simulink model "Phil_VMP_DP_Combo_Task"  (R2013a)
settings: Solver=ode4  SolverMode=SingleTasking  StartTime=0.0  StopTime=inf  FixedStep=BKIN_STEP_TIME  RelTol=1e-3
StartFcn:
  |  warndlg('Dexterit-E models cannot run under simulation. Please compile your model and run it from within Dexterit-E.');set_param(bdroot,'SimulationCommand','stop')
model workspace (MAT data in the model file):
  col_x = 1
  col_y = 2
  RADIUS_VIS = 3
  COLOR_INIT = 4
  START_TARGET_COL = 1
  DELAY_POST_TRIAL_COL = 6
  MAX_REACH_TIME_COL = 4
  DELAY_COL = 5
  BKIN_STEP_TIME = 0.0005
  E_TRIAL_SUCCESS = 8
  SECOND_TARGET_COL = 3
  E_SECOND_TARGET_ON = 4
  WAIT_IN_HOME_COL = 2
  RADIUS_FUNC = 5
  E_SECOND_TARGET_REACHED = 5
  E_TRIAL_FAILURE = 7
  E_NEW_TRIAL = 3
  E_HOME_TARGET_REACHED = 2
  E_SHOW_HOME_TARGET = 6
  LOAD = 1
  TRIAL_TYPE_COL = 7
  RH_LOAD_COL = 8
  Cursor_Diameter_COL = 1
  SPEED_THRESHOLD_START = 2
  GOLDILOCKS = 6
  TOO_FAST = 8
  TOO_SLOW = 7
  LENGTH = 9
  WIDTH = 10
  ROTATION = 11
  SPEED_FEEDBACK_COL = 11
  GOLDILOCKS_COL = 12
  TOO_SLOW_COL = 13
  BASELINE_EEG_COL = 14
  BASELINE_DUR_COL = 15
  E_EEG_BASELINE = 1
  FORCE_CHANNEL_COL = 16
  WALL_WIDTH = 2
  CHANNEL_WIDTH = 3
  VISCOSITY = 4
  E_DEFINE_TRIAL_TYPE = 9
  CHANNEL_LOAD_COL = 17
  HAND_SPEED_THRESHOLD_COL = 18
  E_MOVEMENT_START = 10
  E_BASELINE_END = 11
  ROTATION_ANGLE_COL = 19
  VIS_VS_KIN_COL = 9
  DISTANCE_TO_HOME_COL = 10
  ROTATION_TYPE_COL = 20
  CONST_VISC_FORCE_COL = 21
  VISC_X = 5
  CURL_X = 6
  CURL_Y = 7
  VISC_Y = 8
undefined symbols (not defined in the file): Hand_Feedback, KINARM_DistanceFromTarget, KINARM_general, KINARM_HandInTarget, slselsubs
libraries: xpclib x6, KINARM_EP_loads x4, General x3, Video x3, xpcnilib x1
(part 3 of 3)

== matlab function Phil_VMP_DP_Combo_Task/Visual_Rotation/Triggered Subsystem/Embedded MATLAB Function ==
  settings: fimath=|
      | fimath(...
      | 'RoundMode', 'floor',...
      | 'OverflowMode', 'wrap',...
      | 'ProductMode', 'KeepLSB', 'ProductWordLength', 32,...
      | 'SumMode', 'KeepLSB', 'SumWordLength', 32,...
      | 'CastBeforeSum', false)
  data: rotation output; Trial_Protocol input
function rotation   = Calculate_Desired_Rotation(Trial_Protocol)
% This block supports an embeddable subset of the MATLAB language.
% See the help menu for details. 

%This block was modified by IEB, Sept 24, 2008
%It updates the desired amount of rotation

% NOTE ALL ROTATIONS ARE CURRENTLY IN DEGREES IN THE FUNCTION

% create a persistent variable to remember the rotation amount from one time-step to the next
persistent rotation_memory

if isempty(rotation_memory),            rotation_memory = 0;										end

% where to look in the TP table for these parameters
rotate_type_COL = 20;
rotation_amount_COL = 19;

rotate_type = Trial_Protocol(rotate_type_COL);
rotation_amount = Trial_Protocol(rotation_amount_COL);

if rotate_type == 0
	%set the rotation = 0
	rotation = 0;
elseif rotate_type ==1
	%set the rotation = specified amount
	rotation = rotation_amount;
elseif rotate_type == 2
	%set the rotation to change by specified amount
	rotation = rotation_memory + rotation_amount;
else
	%do nothing
	rotation = rotation_memory;
end

% save the rotation amount for the next time-step
rotation_memory = rotation;

== matlab function Phil_VMP_DP_Combo_Task/Create_MirrorTarget_Table/Embedded MATLAB Mirror Target Table ==
  settings: fimath=|
      | fimath(...
      | 'RoundMode', 'floor',...
      | 'OverflowMode', 'wrap',...
      | 'ProductMode', 'KeepLSB', 'ProductWordLength', 32,...
      | 'SumMode', 'KeepLSB', 'SumWordLength', 32,...
      | 'CastBeforeSum', false)
  data: shoulderXpos input size=2; Mirror_Target_Table output; Target_Table input; Midline_Target_Table output
function [Mirror_Target_Table,Midline_Target_Table]= FMirror_TT(shoulderXpos, Target_Table)
% this function creates a Mirror_Target_Table that is the mirror image of 
% the Target Table, flipped in the X-direction around the subject's midline
% The subject's midline is assumed to be halfway between the two shoulders.

% It also creates a midline Target Table with all targets on the midline.

% all dimensions in m unless otherwise stated
% arguments:
% shoulderXpos: x positions of shoulders (m)
% Target_Table: the complete Target_Table (cm in v1.4)


target_col_x = 1;
center_x = mean(shoulderXpos)*100;				%calculate the subject's midline position (cm)
Mirror_Target_Table = Target_Table;
Midline_Target_Table = Target_Table;

Mirror_Target_Table(:,target_col_x) = 2*center_x-Target_Table(:,target_col_x);
Midline_Target_Table(:,target_col_x) = center_x;

== matlab function Phil_VMP_DP_Combo_Task/Show_Mirror_Target/Embedded MATLAB Function ==
  settings: fimath=|
      | fimath(...
      | 'RoundMode', 'floor',...
      | 'OverflowMode', 'wrap',...
      | 'ProductMode', 'KeepLSB', 'ProductWordLength', 32,...
      | 'SumMode', 'KeepLSB', 'SumWordLength', 32,...
      | 'CastBeforeSum', false)
  data: target input; VCODE output; state input; target_type input; opacity input; target_display input; x_index input; y_index input; num_states input; stateindices input
function VCODE  = fcn(target, state, target_type, opacity, target_display, x_index, y_index, num_states, stateindices)

% VCODEs are length 70. All units in a VCODE should be SI, e.g. (m) and (rad). Elements in a VCODE are defined as follows:
%
% For all target types:
%  1: target type
%       1 - circle
%       2 - ellipse
%       3 - rectangle
%       4 - line
%       5 - triangle
%       11 - circle with label
%       12 - ellipse with label
%       13 - rectangle with label
%       14 - line with label
%       15 - triangle with label
%  2: target on/off status and target display (which display target will appear on)
%		0 - off
%		1 - on, appearing on both subject and operator displays
%       2 - on, appearing on subject display only
%       3 - on, appearing on operator display only
%  3: x position (m)
%  4: y position (m)
%  5: fill colour (RRGGBB) or texture index
%  6: stroke colour (RRGGBB) or texture index
%  7: stroke width
%  8: reserved for target background ID
%  9: opacity
%
% For circles:
%  10: radius (m)
%
% For ellipses:
%  10: major radius (m)
%  11: minor radius (m)
%  12: orientation of major axis (rad)
%
% For rectangles:
%  10: length (m)
%  11: height (m)
%  12: orientation (rad) (relative to x, y already shown)
%
% For lines:
%  10: endpoint x-axis coordinate relative to start point (m)
%  11: endpoint y-axis coordinate relative to start point (m)
%
% For triangles:
%  10: length (m)
%  11: height (m)
%  12: offset of peak from midpoint of length (m)
%  13: orientation (rad)
%
% For all labelled target types:
%  14: reserved
%  15-64: label characters (indexes in ISO 8859-1 character set)
%  65: label colour (0xRRGGBB), opacity is set by the vcode's opacity (9).
%  66: label height (m)
%  67: reserved
%  68: reserved
%  69: reserved
%  70: reserved

VCODE = zeros(1, 70);

% Set the target type.
VCODE(1) = target_type;

% Set the target on/off state. If the state input is 0, the target is off. Users of the VCODE should respect this
% as an indication that the rest of the VCODE will be uninitialized.
if (state <= 0) || (state > num_states)
	VCODE(2) = 0;  % target is off
	return;
else
	VCODE(2) = target_display;  % target is on; target displays as specified by block mask
end

% Set the target position.
VCODE(3) = target(x_index) * 0.01;  % x position (convert from (cm) in target table to (m))
VCODE(4) = target(y_index) * 0.01;  % y position (convert from (cm) in target table to (m))

% Set the fill colour. Fill colour currently comes from the GUI in RRRGGGBBB format.
if stateindices(state, 1) == 0
	VCODE(5) = -2^31;
elseif target(stateindices(state, 1)) < 0
    VCODE(5) = target(stateindices(state, 1));
else
	VCODE(5) = colourshift(target(stateindices(state, 1)));
end

% Set the stroke colour. Stroke colour currently comes from the GUI in RRRGGGBBB format.
if stateindices(state, 2) == 0
	VCODE(6) = -2^31;
elseif target(stateindices(state, 2)) < 0
    VCODE(6) = target(stateindices(state, 2));
else
	VCODE(6) = colourshift(target(stateindices(state, 2)));
end

% Set the stroke width. if target table index for stroke width is zero, then the stroke width is undefined
if stateindices(state, 3) == 0
	VCODE(7) = 0;                   % if stroke width column is 0, then stroke width is 0
elseif stateindices(state, 3) < 0
	VCODE(7) = 0.001;               % if stroke width column is -ve, then a 1mm default is chosen
else
	VCODE(7) = target(stateindices(state, 3)) * 0.01;  % if stroke width column is +ve, convert width from (cm) in target table to (m)
end

% Set the opacity value, clamping it to [0, 100].
if opacity <= 0
    VCODE(9) = 0.0;
elseif opacity >= 100
    VCODE(9) = 100.0;
else
    VCODE(9) = opacity;
end

% Set attributes specific to each target type.
if target_type == 1

    % Handle circle target:
	VCODE(10)=target(stateindices(state, 4)) * 0.01;  % radius (convert from (cm) in target table to (m))

elseif target_type == 2

    % Handle ellipse target:
	VCODE(10) = target(stateindices(state, 4)) * 0.01;  % major radius (convert from (cm) in target table to (m))
	VCODE(11) = target(stateindices(state, 5)) * 0.01;  % minor radius (convert from (cm) in target table to (m))

    if stateindices(state, 6) == 0
		VCODE(12) = 0;  % if orientation column is 0, set orientation to 0 rad
	else
		VCODE(12) = mod(target(stateindices(state, 6)), 360) * pi / 180.0;  % orientation (convert from (degrees) in target table to (rad))
    end

elseif target_type == 3

    % Handle rectangle target:
    VCODE(10) = target(stateindices(state, 4)) * 0.01;  % length (convert from (cm) in target table to (m))
    VCODE(11) = target(stateindices(state, 5)) * 0.01;  % height (convert from (cm) in target table to (m))

    if stateindices(state, 6) == 0
		VCODE(12) = 0;  % if orientation column is 0, set orientation to 0 rad
	else
		VCODE(12) = mod(target(stateindices(state, 6)), 360) * pi / 180.0;  % orientation (convert from (degrees) in target table to (rad))
    end
    
elseif target_type == 4

    % Handle line target:
    VCODE(10) = target(stateindices(state, 4)) * 0.01;  % line endpoint in x axis, relative to start (convert from (cm) in target table to (m))
    VCODE(11) = target(stateindices(state, 5)) * 0.01;  % line endpoint in y axis, relative to start (convert from (cm) in target table to (m))

elseif target_type == 5

    % Handle triangle target:
    VCODE(10) = target(stateindices(state, 4)) * 0.01;  % length (convert from (cm) in target table to (m))

    % If the height column is set to 0 then the triangle is automatically made equilateral, with the base length used as length
    % for all sides. If the height column is non-zero, separate values for height and peak offset are taken from the target table.
    if stateindices(state, 5) == 0
        VCODE(11) = sin(pi / 3.0) * VCODE(10);  % height for equilateral triangle
        VCODE(12) = 0;                          % peak offset for equilateral triangle
    else
        VCODE(11) = target(stateindices(state, 5)) * 0.01;  % height (convert from (cm) in target table to (m))
        VCODE(12) = target(stateindices(state, 6)) * 0.01;  % peak offset (convert from (cm) in target table to (m))
    end

    if stateindices(state, 7) == 0
        VCODE(13) = 0;  % if orientation column is 0, set orientation to 0 rad
    else
        VCODE(13) = mod(target(stateindices(state, 7)), 360) * pi / 180.0;  % orientation (convert from (degrees) in target table to (rad))
    end
end


% The colourshift function converts an "RRRGGGBBB" colour value to RRGBB (as an uint32).
function RRGGBBAA = colourshift(RRRGGGBBB)

blue = cast(mod(RRRGGGBBB, 1000), 'uint32');
green = cast(mod(RRRGGGBBB - blue, 1000000) / 1000, 'uint32');
red = cast((RRRGGGBBB - (green * 1000) - blue) / 1000000, 'uint32');

RRGGBBAA = bitshift(red, 16) + bitshift(green, 8) + blue;

== matlab function Phil_VMP_DP_Combo_Task/KINARM_2ndHandInMirrorTarget/Embedded MATLAB WhichHand ==
  settings: fimath=|
      | fimath(...
      | 'RoundMode', 'floor',...
      | 'OverflowMode', 'wrap',...
      | 'ProductMode', 'KeepLSB', 'ProductWordLength', 32,...
      | 'SumMode', 'KeepLSB', 'SumWordLength', 32,...
      | 'CastBeforeSum', false)
  data: use_dominant_hand input; dominant_hand input; hand output
function hand = WhichHand(use_dominant_hand, dominant_hand)

if use_dominant_hand==1				%use the dominant hand
	hand=dominant_hand;		
else
	hand=3-dominant_hand;			%use the non-dominant hand. i.e. if dominant_hand=2, hand=1 and vice-versa
end

== matlab function Phil_VMP_DP_Combo_Task/KINARM_HandFeedbackInTarget/Embedded MATLAB InsideTarget ==
  settings: fimath=|
      | fimath(...
      | 'RoundMode', 'floor',...
      | 'OverflowMode', 'wrap',...
      | 'ProductMode', 'KeepLSB', 'ProductWordLength', 32,...
      | 'SumMode', 'KeepLSB', 'SumWordLength', 32,...
      | 'CastBeforeSum', false)
  data: handpos input size=2; target_type input; attribcol input; num_targets input; intarget output; Target_Table input
function intarget = FIsInsideTarget(handpos, target_type, attribcol, num_targets, Target_Table)
% all dimensions in m, rad
% arguments:
% handpos: x,y positions of center of target
% attribcol: columns in target table specifying target attributes.  
% Specific to Target_Type
%	circle:
%	[X0,Y0,r...,rn] where:
%	X0,Y0 : centre of circle
%	r : logical radius of circle (i.e. radius used to determine 'in' or 'out' of target)
%	rn: logical radius of other targets (e.g. 2nd, 3rd) also specified in target row.
%   Up to 4 targets can be specified in a row
% ellipse:
%	[X0,Y0,a,b,t...,an, bn, tn] where:
%	X0,Y0 : centre of ellipse
%	a,b : major, minor radii of ellipse
%	t : rotation of ellipse in degrees
%	an,bn : major, minor radii of ellipse of other targets (e.g. 2nd, 3rd) also specified in target row
%	tn : rotation of ellipse in degrees of other targets (e.g. 2nd, 3rd) also specified in target row
%   Up to 4 targets can be specified in a row


target_col_x=1;
target_col_y=2;

x=handpos(1);
y=handpos(2);

intarget = zeros(size(Target_Table,1),4);

X0 = Target_Table(:,target_col_x)*0.01;			%Target Table sizes in cm in v1.4
Y0 = Target_Table(:,target_col_y)*0.01;			%Target Table sizes in cm in v1.4

deltax=x-X0;
deltay=y-Y0;

INT_MAX=2^32-1;

if target_type==1			%circle
	for target=1:num_targets
		r = Target_Table(:,attribcol(target))*0.01;			%Target Table sizes in cm in v1.4
		% simple euclidean distance
		distance2 = deltax.^2 + deltay.^2;					%distance2 is the square of the distance
	    intarget(:,target) = (distance2 <= r.^2);
	end
elseif target_type==2		%ellipse
	for target=1:num_targets
	    a = Target_Table(:,attribcol(target*3-2))*0.01;			%Target Table sizes in cm in v1.4
	    b = Target_Table(:,attribcol(target*3-1))*0.01;			%Target Table sizes in cm in v1.4	
	    t = Target_Table(:,attribcol(target*3))*(pi / 180.0);	%Target Table angles in degrees in v1.4
		sint=sin(t);
		cost=cos(t);
		xrotate=deltax.*cost+deltay.*sint;		%location of x point in ellipse's coordinate frame
		yrotate=-deltax.*sint+deltay.*cost;		%location of y point in ellipse's coordinate frame
		m=yrotate./xrotate;						%slope of line between the (x,y) to (x0,y0) in ellipse's coordinate frame
		y2sq=1./(1./(m.*a).^2+1./b.^2);			%y2sq is y2^2, where y2 is the intersection of the ellipse and the (x,y) to (x0,y0) line
	    intarget(:,target) = (yrotate.^2 <= y2sq);
    end
elseif target_type==3       %rectangle
    for target=1:num_targets
        w = Target_Table(:,attribcol(target*3-2))*0.01;  %width (sizes in cm in v1.4)
        h = Target_Table(:,attribcol(target*3-1))*0.01;  %height (sizes in cm in v1.4)
        
        if attribcol(target*3) > 0
            t = Target_Table(:,attribcol(target*3))*(pi / 180.0);  %angle (angles in degrees in v1.4)
        else
            t = zeros(size(Target_Table, 1), 1);
        end

        sint=sin(t);
        cost=cos(t);

        xrotate=deltax.*cost + deltay.*sint;   %location of x point in rectangle's coordinate frame
        yrotate=-deltax.*sint + deltay.*cost;  %location of y point in rectangle's coordinate frame

        intarget(:,target) = abs(xrotate) <= w/2 & abs(yrotate) <= h/2;
    end
elseif target_type==4       %line
    for target=1:num_targets
        % treat the line like a rectangle of height h and width w
        % determine height (stroke width) in the same fashion as in Show_Target
        if attribcol(target*3-2) == 0                     %0 column index means stroke width of 0
            h = zeros(size(Target_Table, 1), 1);
        elseif attribcol(target*3-2) < 0                  %-ve column index means stroke width of 1mm
            h = ones(size(Target_Table, 1), 1) .* 0.001;
        else
            h = Target_Table(:,attribcol(target*3-2)) * 0.01;  %target table contains width in cm
        end
        
        ex = Target_Table(:,attribcol(target*3-1))*0.01;  %endpoint in x relative to start point (cm)
        ey = Target_Table(:,attribcol(target*3))*0.01;    %endpoint in y relative to start point (cm)
        
        w = sqrt(ex.^2 + ey.^2);                          %width (cm)
        
        % determine the vector from the line's midpoint to the hand position
        handx = deltax - ex/2;
        handy = deltay - ey/2;
        
        t = atan2(ey, ex);                                %calculate angle of the line (rads)
        sint = sin(t);
        cost = cos(t);
        
        xrotate = handx.*cost + handy.*sint;   %location of x point in rectangle's coordinate frame
        yrotate = -handx.*sint + handy.*cost;  %location of y point in rectangle's coordinate frame
 
        intarget(:,target) = abs(xrotate) <= w/2 & abs(yrotate) <= h/2;
    end
elseif target_type==5  % triangle
    for target=1:num_targets
        w = Target_Table(:,attribcol(target*4-3))*0.01;         %length (sizes in cm in v1.4)
        
        % If a height column of 0 is specified, make the triangle equilateral. Otherwise, use the
        % values for height and peak offset from the target table.
        if attribcol(target*4-2) > 0
            h = Target_Table(:,attribcol(target*4-2))*0.01;  %height (sizes in cm in v1.4)
            p = Target_Table(:,attribcol(target*4-1))*0.01;  %peak offset (sizes in cm in v1.4)
        else
            h = w.*sin(pi/3.0);
            p = zeros(size(Target_Table, 1), 1);
        end
        
        if attribcol(target*4) > 0
            t = Target_Table(:,attribcol(target*4))*(pi / 180.0);  %angle (angles in degrees in v1.4)
        else
            t = zeros(size(Target_Table, 1), 1);
        end
        
        sint = sin(t);
        cost = cos(t);
        
        xrotate = deltax.*cost + deltay.*sint;   %location of x point in triangle's coordinate frame
        yrotate = -deltax.*sint + deltay.*cost;  %location of y point in triangle's coordinate frame
        
        % Begin to find centroid of triangle relative to the point on the base beneath the peak. "Left vertex" 
        % refers to the vertex at the left end of the base, and "right vertex" to the vertex at the right end.
        n = w./2.0 + p;  % distance along base from left vertex to peak
        m = w./2.0 - p;  % distance along base from peak to right vertex

        alpha = atan2(h, n);  % angle between base and line from left vertex to peak
        beta = atan2(h, m);   % angle between base and line from right vertex to peak
        
        length1 = sqrt(h.*h + n.*n) ./ 2.0;  % half length of line from left vertex to peak
        length2 = sqrt(h.*h + m.*m) ./ 2.0;  % half length of line from right vertex to peak

        % Determine slope of line from left vertex to midpoint of line from right vertex to peak.
        slope1 = ones(size(Target_Table, 1), 1) .* INT_MAX;
        
        for i=1:size(Target_Table, 1)
            if abs(w(i) - length2(i)*cos(beta(i))) > 0.0
                slope1(i) = length2(i)*sin(beta(i)) / (w(i) - length2(i)*cos(beta(i)));
            end
        end

        % Determine slope of line from right vertex to midpoint of line from left vertex to peak.
        slope2 = ones(size(Target_Table, 1), 1) .* INT_MAX;

        for i=1:size(Target_Table, 1)
            if abs(w(i) - length1(i)*cos(alpha(i))) > 0.0
                slope2(i) = -length1(i)*sin(alpha(i)) / (w(i) - length1(i)*cos(alpha(i)));
            end
        end

        % Calculate centroid position.
        centroid_x = -(m.*slope2 + n.*slope1) ./ (slope1 - slope2);
        centroid_y = slope1.*(centroid_x + n);

        % Test if the point is under the left side of the peak.
        is_under_left = false(size(Target_Table, 1), 1);

        for i=1:size(Target_Table, 1)
            if n(i) >= 0
                is_under_left(i) = (h(i) + (h(i)/n(i)) * (xrotate(i) + centroid_x(i))) >= (yrotate(i) + centroid_y(i));
            else
                is_under_left(i) = (h(i) + (h(i)/n(i)) * (xrotate(i) + centroid_x(i))) <= (yrotate(i) + centroid_y(i));
            end
        end
        
        % Test if the point is under the right side of the peak.
        is_under_right = false(size(Target_Table, 1), 1);

        for i=1:size(Target_Table, 1)
            if m(i) >= 0
                is_under_right(i) = (h(i) - (h(i)/m(i)) * (xrotate(i) + centroid_x(i))) >= (yrotate(i) + centroid_y(i));
            else
                is_under_right(i) = (h(i) - (h(i)/m(i)) * (xrotate(i) + centroid_x(i))) <= (yrotate(i) + centroid_y(i));
            end
        end
        
        intarget(:,target) = is_under_right & ...            %under right side of peak
                             is_under_left & ...             %under left side of peak
                             (yrotate + centroid_y) >= 0.0;  %above base
    end
end

== matlab function Phil_VMP_DP_Combo_Task/KINARM_HandFeedbackInTarget/Embedded MATLAB WhichHand ==
  settings: fimath=|
      | fimath(...
      | 'RoundMode', 'floor',...
      | 'OverflowMode', 'wrap',...
      | 'ProductMode', 'KeepLSB', 'ProductWordLength', 32,...
      | 'SumMode', 'KeepLSB', 'SumWordLength', 32,...
      | 'CastBeforeSum', false)
  data: use_dominant_hand input; dominant_hand input; hand output; cursor output
function [hand, cursor] = WhichHand(use_dominant_hand, dominant_hand)

if use_dominant_hand==1				%use the dominant hand
	hand=dominant_hand;		
	cursor = 1;
else
	hand=3-dominant_hand;			%use the non-dominant hand. i.e. if dominant_hand=2, hand=1 and vice-versa
	cursor = 2;
end

== matlab function Phil_VMP_DP_Combo_Task/Visual vs. Kinesthetic Selector/MATLAB Function ==
  data: Trial_Protocol input; y output; distance_from_target input; reachingOut input
function y = visVkin(Trial_Protocol, distance_from_target, reachingOut)
%#codegen
%This function generates a constant depending on whether or not the trial
%is to be visual or kinesthetic AND how far the non-dominant hand is from
%the non-dominant home target position.

%constant will be sent into Hand_Feedback1 (non-active hand)

%Made by ATB 2/27/15
vis_vs_kin_COL = 9;        % find the boolean for visual or kin
distance_to_home_COL = 10;  % find the distance threshold column

vis_OR_kin = Trial_Protocol(vis_vs_kin_COL); % 0=visual, 1=kinesthetic
dist_to_home_threshold = Trial_Protocol(distance_to_home_COL)*0.01; %distance(cm) threshold for when to turn back on the visual feedback
dist_to_home = distance_from_target(2); % selects the distance from cursor to 2nd row target (home)

u = 2; %set default to show non-dominant hand

if vis_OR_kin == 0
    u = 2;              % show non-dom hand
elseif vis_OR_kin == 1
    if dist_to_home <= dist_to_home_threshold && reachingOut == 0
        u = 2;
    elseif dist_to_home <= dist_to_home_threshold && reachingOut == 1
        u = 0;
    elseif dist_to_home > dist_to_home_threshold
        u = 0;
    end
end

y = u;      % output the feedback_status

== matlab function Phil_VMP_DP_Combo_Task/KINARM_DistanceFromMirrorTarget/Embedded MATLAB InsideTarget ==
  settings: fimath=|
      | fimath(...
      | 'RoundMode', 'floor',...
      | 'OverflowMode', 'wrap',...
      | 'ProductMode', 'KeepLSB', 'ProductWordLength', 32,...
      | 'SumMode', 'KeepLSB', 'SumWordLength', 32,...
      | 'CastBeforeSum', false)
  data: handpos input size=2; distance output; Target_Table input
function distance = Distance(handpos, Target_Table)
% all dimensions in m, rad
% arguments:
% handpos: x,y positions of center of target

target_col_x=1;
target_col_y=2;
x=handpos(1);
y=handpos(2);

X0 = Target_Table(:,target_col_x)*(-0.01);      %Target Table sizes in cm in v1.4
Y0 = Target_Table(:,target_col_y)*0.01;			%Target Table sizes in cm in v1.4

distance = sqrt( (X0 - x).^2 + (Y0 - y).^2 );

== matlab function Phil_VMP_DP_Combo_Task/KINARM_DistanceFromMirrorTarget/Embedded MATLAB WhichHand ==
  settings: fimath=|
      | fimath(...
      | 'RoundMode', 'floor',...
      | 'OverflowMode', 'wrap',...
      | 'ProductMode', 'KeepLSB', 'ProductWordLength', 32,...
      | 'SumMode', 'KeepLSB', 'SumWordLength', 32,...
      | 'CastBeforeSum', false)
  data: use_dominant_hand input; dominant_hand input; hand output
function hand = WhichHand(use_dominant_hand, dominant_hand)

if use_dominant_hand==1				%use the dominant hand
	hand=dominant_hand;		
else
	hand=3-dominant_hand;			%use the non-dominant hand. i.e. if dominant_hand=2, hand=1 and vice-versa
end

== matlab function Phil_VMP_DP_Combo_Task/Visual_Rotation/Dom Trail ==
  data: handFeedbackVcode input; VCODETrail output
function VCODETrail = makeTrail(handFeedbackVcode)
%#create a permanent variable that will exist in between calls to this method.
  persistent trail
  persistent ignoreCounter

  if isempty(trail)
    %this will leave behind the last 10 positions, adjust this as required.
    trail  = zeros(10, 70);
    ignoreCounter = 40; %ensure we record the first VCode
  end

  %this will ensure we only grab each 40th VCode. The model runs at 2KHz,
  %so if we don't do this then there will just be a solid trail of VCodes where you
  %can't see between any of them. You can adjust this number as required!
  if ignoreCounter < 40
    ignoreCounter = ignoreCounter + 1;
    VCODETrail = trail;
    return;
  end

  %reset the counter so the above if statement still works
  ignoreCounter = 0;
  %This will help fade out the older VCodes
  opacityChange = 100.0/  size(trail,1);
  opacity = opacityChange;

  %Move each VCode one position down the list.
  for row=size(trail,1):-1:2
    trail(row,:) = trail(row-1,:);

    %#This code changes the opacity of the VCode and therefore fades it out.
    trail(row, 9) = opacity;
    opacity = opacity + opacityChange;
  end

  trail(1,:) = handFeedbackVcode(1,:);
  VCODETrail = trail;

== matlab function Phil_VMP_DP_Combo_Task/Hand_Feedback1/FeedFwdArm ==
  settings: fimath=|
      | fimath(...
      | 'RoundMode', 'floor',...
      | 'OverflowMode', 'wrap',...
      | 'ProductMode', 'KeepLSB', 'ProductWordLength', 32,...
      | 'SumMode', 'KeepLSB', 'SumWordLength', 32,...
      | 'CastBeforeSum', false)
  data: KINARMdata input; VCODES_in input; VCODES_out output; fdbk_stts_mdl input; block_settings input; Task_Wide_Parameters input
function VCODES_out  = fcn(KINARMdata,VCODES_in,fdbk_stts_mdl, block_settings, Task_Wide_Parameters)
%
% This function creates the VCODEs for the hand position feedback for both
% hands.  Various options in the Mask of the Simulink block in which this
% embedded Matlab file sits, allow the user to specify how often
% the hand feedback is updated as well as the source of the style and status
% of the hand feedback.  
%
% block_settings is the value chosen by the user in the Mask for parent Simulink
% block.  Note: that even if the block is wired up to accept Task Program 
% control of hand feedback style and status, this embedded Matlab file allows
% the GUI to over-ride those settings.  However, if the GUI requests that
% the parent block use Task Program control for the style and/or status when
% it has not been programmed in, then this embedded Matlab file handles this
% appropriately and ignore the request for Task Program control.  
%
% block_settings=1 -- parent block does not have any Task Program control over style or status
% block_settings=2 -- parent block has Task Program control over status only
% block_settings=3 -- parent block has Task Program control over both style and status
%
% fdbk_stts_mdl (only potentially used if block_settings=2) 
% fdbk_stts_mdl=0 -- neither hand on
% fdbk_stts_mdl=1 -- dominant hand on
% fdbk_stts_mdl=2 -- non-dominant hand on
% fdbk_stts_mdl=3 -- both hands on
%
% VCODES (only potentially used if block_settings=3) 
% VCODES for dominant and non-dominant, input to parent block 
Cursor_Diameter_COL = 1;

dominant_arm=KINARMdata(3,1);
feedfwd=KINARMdata(3,2);				%amount of feedforward extrapolation for hand position(s)
fdbk_stts_GUI=KINARMdata(3,3);			%status of hand feedback requested from GUI
fdbk_src_GUI=KINARMdata(3,4);			%source of hand feedback style requested from GUI
fdbk_clr_GUI=KINARMdata(3,5);			%colour of hand feedback required by GUI
fdbk_radius_GUI=KINARMdata(3,6).*Task_Wide_Parameters(Cursor_Diameter_COL);		%radius of hand feedback required by GUI


%----------------Feedback Style ----------------
% IF GUI asks for feedback style from Task Program (fdbk_src_GUI==0)
% AND if Task Program has been chosen to supply feedback style (block_settings==3)
% AND if Task Program actually supplies appropriate feedback styles (size(VCODES_in,2)==70)
if fdbk_src_GUI==0 && block_settings==3 && size(VCODES_in,2)==70
    VCODES=VCODES_in;
else
    VCODES=zeros(2,70);						%set default
	VCODES(:,1)=1;							%target_type of circle
	VCODES(:,5)=fdbk_clr_GUI;				%fill colour as specified by GUI
	VCODES(:,6)=fdbk_clr_GUI;				%stroke colour same as fill colour
	VCODES(:,7)=0;							%no stroke width
    VCODES(:,9)=100.0;                      %100% opacity
	VCODES(:,10)=fdbk_radius_GUI;			%radius (m) as specified by GUI
end

%----------------Feedback Status ----------------
%feedback status from GUI sets the default to be used
feedback_status=fdbk_stts_GUI;


if fdbk_stts_GUI==4				%if GUI has requested Task Program control of feedback status
	if block_settings==2		%if there is Task Program control ONLY of status (but not style)
		feedback_status=fdbk_stts_mdl;		%then use feedback status input from parent block
	elseif block_settings==3	%if there is Task Program control of both status and style
		feedback_status=4;		%then let the input VCODEs handle the status
	else						%otherwise assume that the Task Program did not provide style OR status
		feedback_status=3;		%then set both hands are always on as a default
    end
else		%if GUI is controlling feedback status
	feedback_status=fdbk_stts_GUI;
end

%set the status of the hand-feedback in the VCODES
switch feedback_status
	case 0					%show neither hand feedback
		VCODES(1,2)=0;
		VCODES(2,2)=0;
	case 1					%show ONLY dominant hand feedback
		VCODES(1,2)=1;
		VCODES(2,2)=0;
	case 2					%show ONLY non-dominant hand feedback
		VCODES(1,2)=0;
		VCODES(2,2)=1;
	case 4					%VCODES already control hand feedback
		%do nothing
	otherwise				%show both hand feedbacks
		VCODES(1,2)=1;
		VCODES(2,2)=1;
end

%----------------Feedback Position ----------------
%set the position of the hand feedback.
for i=1:2
	if i==1
		active_arm=KINARMdata(3,1);			%choose dominant arm first
	else
		active_arm=3-KINARMdata(3,1);		%choose non-dominant arm 2nd
	end
	HandXPos=KINARMdata(active_arm,23);		%(m)
	HandYPos=KINARMdata(active_arm,24);		%(m)
	HandXVel=KINARMdata(active_arm,25);		%(m/s)
	HandYVel=KINARMdata(active_arm,26);		%(m/s)

	% feed-forward hand position (m)
	HandXPos_ff = HandXPos + HandXVel*feedfwd;
	HandYPos_ff = HandYPos + HandYVel*feedfwd;
	VCODES(i,3)=HandXPos_ff;				%target position in m 
	VCODES(i,4)=HandYPos_ff;				%target position in m 
end

VCODES_out=VCODES;

== matlab function Phil_VMP_DP_Combo_Task/Hand_Feedback/FeedFwdArm ==
  settings: fimath=|
      | fimath(...
      | 'RoundMode', 'floor',...
      | 'OverflowMode', 'wrap',...
      | 'ProductMode', 'KeepLSB', 'ProductWordLength', 32,...
      | 'SumMode', 'KeepLSB', 'SumWordLength', 32,...
      | 'CastBeforeSum', false)
  data: KINARMdata input; VCODES_in input; VCODES_out output; fdbk_stts_mdl input; block_settings input; Task_Wide_Parameters input
function VCODES_out  = fcn(KINARMdata,VCODES_in,fdbk_stts_mdl, block_settings, Task_Wide_Parameters)
%
% This function creates the VCODEs for the hand position feedback for both
% hands.  Various options in the Mask of the Simulink block in which this
% embedded Matlab file sits, allow the user to specify how often
% the hand feedback is updated as well as the source of the style and status
% of the hand feedback.  
%
% block_settings is the value chosen by the user in the Mask for parent Simulink
% block.  Note: that even if the block is wired up to accept Task Program 
% control of hand feedback style and status, this embedded Matlab file allows
% the GUI to over-ride those settings.  However, if the GUI requests that
% the parent block use Task Program control for the style and/or status when
% it has not been programmed in, then this embedded Matlab file handles this
% appropriately and ignore the request for Task Program control.  
%
% block_settings=1 -- parent block does not have any Task Program control over style or status
% block_settings=2 -- parent block has Task Program control over status only
% block_settings=3 -- parent block has Task Program control over both style and status
%
% fdbk_stts_mdl (only potentially used if block_settings=2) 
% fdbk_stts_mdl=0 -- neither hand on
% fdbk_stts_mdl=1 -- dominant hand on
% fdbk_stts_mdl=2 -- non-dominant hand on
% fdbk_stts_mdl=3 -- both hands on
%
% VCODES (only potentially used if block_settings=3) 
% VCODES for dominant and non-dominant, input to parent block 
Cursor_Diameter_COL = 1;

dominant_arm=KINARMdata(3,1);
feedfwd=KINARMdata(3,2);				%amount of feedforward extrapolation for hand position(s)
fdbk_stts_GUI=KINARMdata(3,3);			%status of hand feedback requested from GUI
fdbk_src_GUI=KINARMdata(3,4);			%source of hand feedback style requested from GUI
fdbk_clr_GUI=KINARMdata(3,5);			%colour of hand feedback required by GUI
fdbk_radius_GUI=KINARMdata(3,6).*Task_Wide_Parameters(Cursor_Diameter_COL);		%radius of hand feedback required by GUI


%----------------Feedback Style ----------------
% IF GUI asks for feedback style from Task Program (fdbk_src_GUI==0)
% AND if Task Program has been chosen to supply feedback style (block_settings==3)
% AND if Task Program actually supplies appropriate feedback styles (size(VCODES_in,2)==70)
if fdbk_src_GUI==0 && block_settings==3 && size(VCODES_in,2)==70
    VCODES=VCODES_in;
else
    VCODES=zeros(2,70);						%set default
	VCODES(:,1)=1;							%target_type of circle
	VCODES(:,5)=fdbk_clr_GUI;				%fill colour as specified by GUI
	VCODES(:,6)=fdbk_clr_GUI;				%stroke colour same as fill colour
	VCODES(:,7)=0;							%no stroke width
    VCODES(:,9)=100.0;                      %100% opacity
	VCODES(:,10)=fdbk_radius_GUI;			%radius (m) as specified by GUI
end

%----------------Feedback Status ----------------
%feedback status from GUI sets the default to be used
feedback_status=fdbk_stts_GUI;


if fdbk_stts_GUI==4				%if GUI has requested Task Program control of feedback status
	if block_settings==2		%if there is Task Program control ONLY of status (but not style)
		feedback_status=fdbk_stts_mdl;		%then use feedback status input from parent block
	elseif block_settings==3	%if there is Task Program control of both status and style
		feedback_status=4;		%then let the input VCODEs handle the status
	else						%otherwise assume that the Task Program did not provide style OR status
		feedback_status=3;		%then set both hands are always on as a default
    end
else		%if GUI is controlling feedback status
	feedback_status=fdbk_stts_GUI;
end

%set the status of the hand-feedback in the VCODES
switch feedback_status
	case 0					%show neither hand feedback
		VCODES(1,2)=0;
		VCODES(2,2)=0;
	case 1					%show ONLY dominant hand feedback
		VCODES(1,2)=1;
		VCODES(2,2)=0;
	case 2					%show ONLY non-dominant hand feedback
		VCODES(1,2)=0;
		VCODES(2,2)=1;
	case 4					%VCODES already control hand feedback
		%do nothing
	otherwise				%show both hand feedbacks
		VCODES(1,2)=1;
		VCODES(2,2)=1;
end

%----------------Feedback Position ----------------
%set the position of the hand feedback.
for i=1:2
	if i==1
		active_arm=KINARMdata(3,1);			%choose dominant arm first
	else
		active_arm=3-KINARMdata(3,1);		%choose non-dominant arm 2nd
	end
	HandXPos=KINARMdata(active_arm,23);		%(m)
	HandYPos=KINARMdata(active_arm,24);		%(m)
	HandXVel=KINARMdata(active_arm,25);		%(m/s)
	HandYVel=KINARMdata(active_arm,26);		%(m/s)

	% feed-forward hand position (m)
	HandXPos_ff = HandXPos + HandXVel*feedfwd;
	HandYPos_ff = HandYPos + HandYVel*feedfwd;
	VCODES(i,3)=HandXPos_ff;				%target position in m 
	VCODES(i,4)=HandYPos_ff;				%target position in m 
end

VCODES_out=VCODES;

== matlab function Phil_VMP_DP_Combo_Task/Force Channel/Calculate force channel ==
  data: target1 input; forces output; target2 input; xIdx input; yIdx input; KINData input; loadTable input; enable_forces input
function forces = forceChannel(target1, target2, xIdx, yIdx, KINData, loadTable, enable_forces)

	persistent lastForcesEnabledValue forceEnableTime clockCycle outsideChannel lastHandPosition;
	
	if isempty(lastForcesEnabledValue), lastForcesEnabledValue = 0;		end
	if isempty(forceEnableTime),        forceEnableTime = 1;			end
	if isempty(clockCycle),				clockCycle = 0;					end
	if isempty(outsideChannel),			outsideChannel = 0;				end
	if isempty(lastHandPosition),		lastHandPosition = zeros(1,2);	end


	%we need to keep track of the time so we can safely ramp up forces when 
	%the trial starts.
	clockCycle = clockCycle + 1;
	if lastForcesEnabledValue == 0 && enable_forces == 1
		forceEnableTime = clockCycle;
	end

	lastForcesEnabledValue = enable_forces;

	%start out assuming we will apply no forces.
	forces = zeros(1, 4);

	channelWidthM = abs((loadTable(3) * 0.01) / 2.0);%get the width of the zero force zone and convert to meters
	wallWidthM = abs(loadTable(2) * 0.01);			%get the width of the wall where forces cut out and convert to meters.
	wallStiffness = abs(loadTable(1));				%in N/m
	viscosity = -abs(loadTable(4));					%in N/(m/s)

	active_arm=KINData(3,1);			%choose dominant arm first
    active_arm = 3-active_arm;          %switch to inactive arm
	xHand=KINData(active_arm,23);		%(m)
	yHand=KINData(active_arm,24);		%(m)

	%get the target positions and convert them to meters. These are pulled
	%from the VCODES. Positions 3 and 4 are x and y, respectively
	x1 = target1(3);
	y1 = target1(4);
	x2 = target2(3);
	y2 = target2(4);

	%http://www.codeguru.com/forum/showthread.php?threadid=194400
	%This calculations gives us the distance away from the line we are now.
	distToLine = abs(((x2 - x1)*(y1-yHand)) - ((x1 - xHand)*(y2-y1))) / sqrt( (x2 - x1)^2 + (y2 - y1)^2 );

	HXVEL_index = 25;			% Hand x velocity
	HYVEL_index = 26;			% Hand y velocity
	HXVEL = KINData( active_arm, HXVEL_index );
	HYVEL = KINData( active_arm, HYVEL_index );
	viscosityX = HXVEL * viscosity;
	viscosityY = HYVEL * viscosity;

	%we only ever want to provide a viscous load perpendicular to
	%the force channel. This viscous force will be used to dampen
	%any instability.
	if (x2 == x1) %infinite slope
		viscosityY = 0;	
	elseif (y2 == y1) %0 slope
		viscosityX = 0;
	else
		m = (y2 - y1) / (x2 - x1);
		perpM = -(1/m);	

		%we need to scale the viscous load to only the components
		%that are perpendicular to the line. To do that we find the 
		%projection of the velocity vecotor on a line perpendicular to the
		%force channel
		perpVect = [1 perpM];
		perpUnitVector = perpVect / norm(perpVect);

		%this finds the projection of the vector perpendicular to the channel
		dotProduct = dot([viscosityX viscosityY], perpUnitVector);
		scaledForces = dotProduct * perpUnitVector;

		viscosityX = scaledForces(1);
		viscosityY = scaledForces(2);
	end

	%forces 1,2 are for right arm, 3,4 are for left
	addIdx = 0;
	if active_arm == 2
		addIdx = 2;
	end

	% if we are outside the force wall we need to make sure we don't turn it
	%back on until we are in the channel. Otherwise it's quite jarring to be pulled in.
	if distToLine > (wallWidthM + channelWidthM)
		outsideChannel = 1;
		return
	elseif enable_forces == 0
		return	
	%if we are in the force channel we still need to viscous loads to aid in stability
	%if we are bouncing between the walls. 
	elseif distToLine < channelWidthM 
		outsideChannel = 0; %we're in the channel, so we can turn forces back on if they were off.
		return
	elseif outsideChannel == 1    
		%If we were outside the wall then forces are all off. We only want to turn
		%forces back on if the hand has crossed the line of the force channel, that way
		%you are not pushed into the channel, it only feels like you hit a wall.
		%By looking at the previous hand position and the current hand position
		%we can see if that line segment crosses the channel line, in which case we can
		%turn the forces back on.
		if doLinesIntersect([x1 y1], [x2 y2], [xHand yHand], lastHandPosition) == 1
			outsideChannel = 0;
		else
			return
		end
	end

	distIntoWall = distToLine - channelWidthM;

	if (x2 == x1) %all force wille be in x direction
		y = 0;
		if xHand < x1
			x = distIntoWall;
		else
			x = -distIntoWall;
		end
	elseif (y2 == y1) %all force will be in Y direction
		x = 0;
		if yHand < y1
			y = distIntoWall;
		else
			y = -distIntoWall;
		end	
	else
		%we need to find out how far off the line in X and Y we are in meters so 
		%we can properly convert the wall stiffness in N/m to a force.
		m = (y2 - y1) / (x2 - x1);
		b = y1 - (m * x1);

		perpM = -(1/m);	
		perpB = yHand - (perpM * xHand);

		xIntersect = (b - perpB) / (perpM - m);
		yIntersect = (m * xIntersect) + b;

		%x and y are converted to distances in meters from the center line
		x = xIntersect - xHand;
		y = yIntersect - yHand;

		%take the distances from center and convert to a unit vector,
		%then multiply by the distance to where the forces start
		%this gives us a clean number to use when calculating wall force.
		x = (x / sqrt(x^2 + y^2)) * distIntoWall;
		y = (y / sqrt(x^2 + y^2)) * distIntoWall;
	end

	%we don't want to just shut off the forces, we need to ramp them down
	%somewhat. This finds out how far into the wall we are and allows us
	%to ramp down the forces over the last 25% of the wll.
	forceRampDownZoneSizePercent = 0.75; %start ramping down the forces in the last 25% of the wall
	forceMaxEndLocInWallM = forceRampDownZoneSizePercent * wallWidthM;
	distanceIntoWall = distToLine - channelWidthM;
	scaleWallForce = 1; %assume we can run at full calculated wall force

	if distanceIntoWall > forceMaxEndLocInWallM   %we are in the ramp down zone
		distIntoRampDownZone = distanceIntoWall - forceMaxEndLocInWallM;
		rampDownZoneWidth = wallWidthM  - forceMaxEndLocInWallM;
		scaleWallForce = (rampDownZoneWidth - distIntoRampDownZone) / rampDownZoneWidth;
	end

	%within the first 1.5 seconds of the trial we don't wan to jar anyone
	%this ramps the forces up slowly so you get a gentle nudge into
	%the force channel, not a violent jerk.
	timeDelta = clockCycle - forceEnableTime;
	timeScaling = 1;
	if (timeDelta < 1500)
		timeScaling = timeDelta / 1500.0;
	end

	%the final forces will be wall force + viscous.
	forces(addIdx + 1) = (wallStiffness * scaleWallForce * timeScaling * x) + viscosityX;
	forces(addIdx + 2) = (wallStiffness * scaleWallForce  * timeScaling * y) + viscosityY;

	lastHandPosition(1) = xHand;
	lastHandPosition(2) = yHand;
end

function bIntersect = doLinesIntersect(Ap1, Ap2, Bp1, Bp2)
    %This method for finding out if 2 lines segements intersect comes from:
    %http://stackoverflow.com/questions/563198/how-do-you-detect-where-two-line-segments-intersect
   	e = Ap2-Ap1;
    f = Bp2-Bp1;
    p = [-e(2) e(1)];
    h = dot((Ap1 - Bp1), p) / dot (f, p);
    
    if h >=0 && h <= 1
        bIntersect = 1;
    else
        bIntersect = 0;
    end
end

== matlab function Phil_VMP_DP_Combo_Task/Show_Mirror_Target1/Embedded MATLAB Function ==
  settings: fimath=|
      | fimath(...
      | 'RoundMode', 'floor',...
      | 'OverflowMode', 'wrap',...
      | 'ProductMode', 'KeepLSB', 'ProductWordLength', 32,...
      | 'SumMode', 'KeepLSB', 'SumWordLength', 32,...
      | 'CastBeforeSum', false)
  data: target input; VCODE output; state input; target_type input; opacity input; target_display input; x_index input; y_index input; num_states input; stateindices input
function VCODE  = fcn(target, state, target_type, opacity, target_display, x_index, y_index, num_states, stateindices)

% VCODEs are length 70. All units in a VCODE should be SI, e.g. (m) and (rad). Elements in a VCODE are defined as follows:
%
% For all target types:
%  1: target type
%       1 - circle
%       2 - ellipse
%       3 - rectangle
%       4 - line
%       5 - triangle
%       11 - circle with label
%       12 - ellipse with label
%       13 - rectangle with label
%       14 - line with label
%       15 - triangle with label
%  2: target on/off status and target display (which display target will appear on)
%		0 - off
%		1 - on, appearing on both subject and operator displays
%       2 - on, appearing on subject display only
%       3 - on, appearing on operator display only
%  3: x position (m)
%  4: y position (m)
%  5: fill colour (RRGGBB) or texture index
%  6: stroke colour (RRGGBB) or texture index
%  7: stroke width
%  8: reserved for target background ID
%  9: opacity
%
% For circles:
%  10: radius (m)
%
% For ellipses:
%  10: major radius (m)
%  11: minor radius (m)
%  12: orientation of major axis (rad)
%
% For rectangles:
%  10: length (m)
%  11: height (m)
%  12: orientation (rad) (relative to x, y already shown)
%
% For lines:
%  10: endpoint x-axis coordinate relative to start point (m)
%  11: endpoint y-axis coordinate relative to start point (m)
%
% For triangles:
%  10: length (m)
%  11: height (m)
%  12: offset of peak from midpoint of length (m)
%  13: orientation (rad)
%
% For all labelled target types:
%  14: reserved
%  15-64: label characters (indexes in ISO 8859-1 character set)
%  65: label colour (0xRRGGBB), opacity is set by the vcode's opacity (9).
%  66: label height (m)
%  67: reserved
%  68: reserved
%  69: reserved
%  70: reserved

VCODE = zeros(1, 70);

% Set the target type.
VCODE(1) = target_type;

% Set the target on/off state. If the state input is 0, the target is off. Users of the VCODE should respect this
% as an indication that the rest of the VCODE will be uninitialized.
if (state <= 0) || (state > num_states)
	VCODE(2) = 0;  % target is off
	return;
else
	VCODE(2) = target_display;  % target is on; target displays as specified by block mask
end

% Set the target position.
VCODE(3) = target(x_index) * 0.01;  % x position (convert from (cm) in target table to (m))
VCODE(4) = target(y_index) * 0.01;  % y position (convert from (cm) in target table to (m))

% Set the fill colour. Fill colour currently comes from the GUI in RRRGGGBBB format.
if stateindices(state, 1) == 0
	VCODE(5) = -2^31;
elseif target(stateindices(state, 1)) < 0
    VCODE(5) = target(stateindices(state, 1));
else
	VCODE(5) = colourshift(target(stateindices(state, 1)));
end

% Set the stroke colour. Stroke colour currently comes from the GUI in RRRGGGBBB format.
if stateindices(state, 2) == 0
	VCODE(6) = -2^31;
elseif target(stateindices(state, 2)) < 0
    VCODE(6) = target(stateindices(state, 2));
else
	VCODE(6) = colourshift(target(stateindices(state, 2)));
end

% Set the stroke width. if target table index for stroke width is zero, then the stroke width is undefined
if stateindices(state, 3) == 0
	VCODE(7) = 0;                   % if stroke width column is 0, then stroke width is 0
elseif stateindices(state, 3) < 0
	VCODE(7) = 0.001;               % if stroke width column is -ve, then a 1mm default is chosen
else
	VCODE(7) = target(stateindices(state, 3)) * 0.01;  % if stroke width column is +ve, convert width from (cm) in target table to (m)
end

% Set the opacity value, clamping it to [0, 100].
if opacity <= 0
    VCODE(9) = 0.0;
elseif opacity >= 100
    VCODE(9) = 100.0;
else
    VCODE(9) = opacity;
end

% Set attributes specific to each target type.
if target_type == 1

    % Handle circle target:
	VCODE(10)=target(stateindices(state, 4)) * 0.01;  % radius (convert from (cm) in target table to (m))

elseif target_type == 2

    % Handle ellipse target:
	VCODE(10) = target(stateindices(state, 4)) * 0.01;  % major radius (convert from (cm) in target table to (m))
	VCODE(11) = target(stateindices(state, 5)) * 0.01;  % minor radius (convert from (cm) in target table to (m))

    if stateindices(state, 6) == 0
		VCODE(12) = 0;  % if orientation column is 0, set orientation to 0 rad
	else
		VCODE(12) = mod(target(stateindices(state, 6)), 360) * pi / 180.0;  % orientation (convert from (degrees) in target table to (rad))
    end

elseif target_type == 3

    % Handle rectangle target:
    VCODE(10) = target(stateindices(state, 4)) * 0.01;  % length (convert from (cm) in target table to (m))
    VCODE(11) = target(stateindices(state, 5)) * 0.01;  % height (convert from (cm) in target table to (m))

    if stateindices(state, 6) == 0
		VCODE(12) = 0;  % if orientation column is 0, set orientation to 0 rad
	else
		VCODE(12) = mod(target(stateindices(state, 6)), 360) * pi / 180.0;  % orientation (convert from (degrees) in target table to (rad))
    end
    
elseif target_type == 4

    % Handle line target:
    VCODE(10) = target(stateindices(state, 4)) * 0.01;  % line endpoint in x axis, relative to start (convert from (cm) in target table to (m))
    VCODE(11) = target(stateindices(state, 5)) * 0.01;  % line endpoint in y axis, relative to start (convert from (cm) in target table to (m))

elseif target_type == 5

    % Handle triangle target:
    VCODE(10) = target(stateindices(state, 4)) * 0.01;  % length (convert from (cm) in target table to (m))

    % If the height column is set to 0 then the triangle is automatically made equilateral, with the base length used as length
    % for all sides. If the height column is non-zero, separate values for height and peak offset are taken from the target table.
    if stateindices(state, 5) == 0
        VCODE(11) = sin(pi / 3.0) * VCODE(10);  % height for equilateral triangle
        VCODE(12) = 0;                          % peak offset for equilateral triangle
    else
        VCODE(11) = target(stateindices(state, 5)) * 0.01;  % height (convert from (cm) in target table to (m))
        VCODE(12) = target(stateindices(state, 6)) * 0.01;  % peak offset (convert from (cm) in target table to (m))
    end

    if stateindices(state, 7) == 0
        VCODE(13) = 0;  % if orientation column is 0, set orientation to 0 rad
    else
        VCODE(13) = mod(target(stateindices(state, 7)), 360) * pi / 180.0;  % orientation (convert from (degrees) in target table to (rad))
    end
end


% The colourshift function converts an "RRRGGGBBB" colour value to RRGBB (as an uint32).
function RRGGBBAA = colourshift(RRRGGGBBB)

blue = cast(mod(RRRGGGBBB, 1000), 'uint32');
green = cast(mod(RRRGGGBBB - blue, 1000000) / 1000, 'uint32');
red = cast((RRRGGGBBB - (green * 1000) - blue) / 1000000, 'uint32');

RRGGBBAA = bitshift(red, 16) + bitshift(green, 8) + blue;
